simulink model "Laboratorio3CasoA1"  (R2023a)
settings: Solver=VariableStepAuto  StartTime=0.0  StopTime=3/Frecuencia  RelTol=1e-3
undefined symbols (not defined in the file): LCarga, LLinea, RCarga, RLLinea, VSPeak, VSRms
libraries: spsPowerLib x6, spsSeriesRLCBranchLib x4, spsMultimeterLib x2, spsLinearTransformerLib x2, spsACVoltageSourceLib x2, spspowerguiLib x1
settings Model: Creator=mluser  LastModifiedBy=USUARIO
settings OptimizationCC: ReuseModelBlockBuffer=off

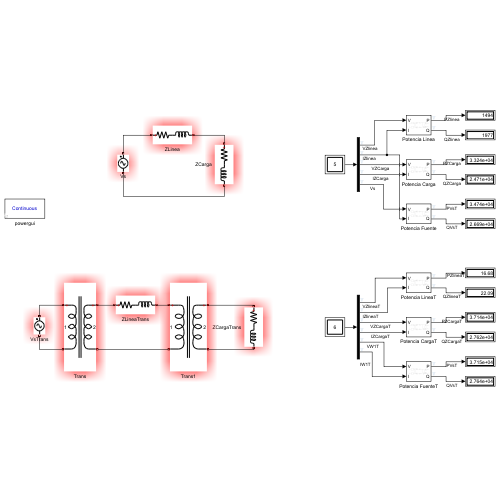
[thumbnail: Simulink's stored preview of the top-level diagram]
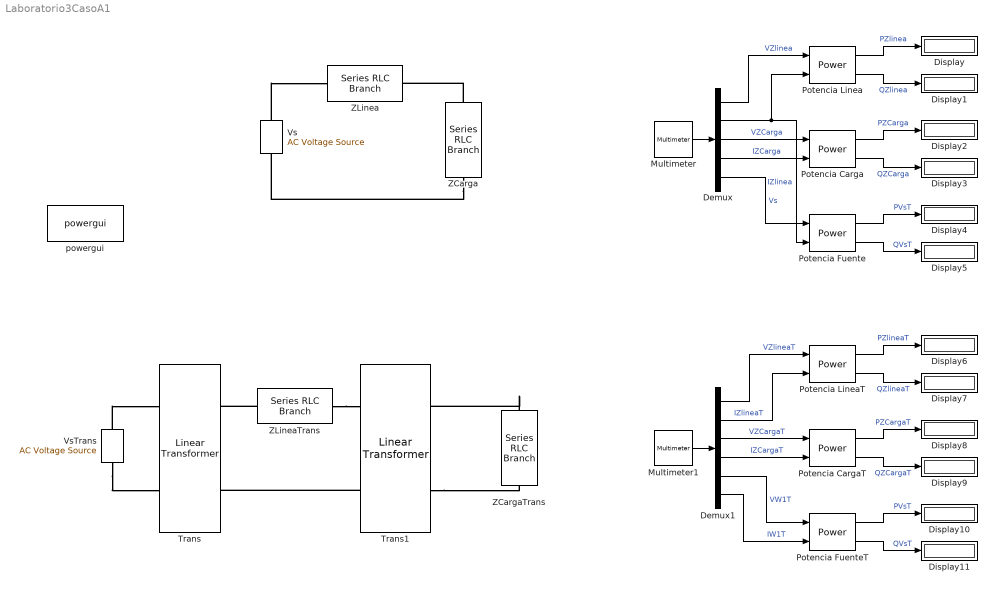
== system Laboratorio3CasoA1 ==
  Demux : Demux  Outputs=5
  Demux1 : Demux  Outputs=6
  Display{,1..11} (12 alike) : Display
  Multimeter : spsMultimeterLib/Multimeter  L=24  sel=[3 13 1 11 9]  yselected={}  Gain=[1 1 1 1 1]  OutputType=Complex  PlotAtSimulationStop=off  PhasorSimulation=off
  Multimeter1 : spsMultimeterLib/Multimeter  L=24  sel=[4 14 2 12 5 15]  yselected={}  Gain=[1 1 1 1 1 1]  OutputType=Complex  PlotAtSimulationStop=off  PhasorSimulation=off
  Potencia Carga : spsPowerLib/Power  Freq=Frecuencia  Vinit=[1, 0]  Iinit=[1, 0]  Ts=0
  Potencia CargaT : spsPowerLib/Power  Freq=Frecuencia  Vinit=[1, 0]  Iinit=[1, 0]  Ts=0
  Potencia Fuente : spsPowerLib/Power  Freq=Frecuencia  Vinit=[1, 0]  Iinit=[1, 0]  Ts=0
  Potencia FuenteT : spsPowerLib/Power  Freq=Frecuencia  Vinit=[1, 0]  Iinit=[1, 0]  Ts=0
  Potencia Linea : spsPowerLib/Power  Freq=Frecuencia  Vinit=[1, 0]  Iinit=[1, 0]  Ts=0
  Potencia LineaT : spsPowerLib/Power  Freq=Frecuencia  Vinit=[1, 0]  Iinit=[1, 0]  Ts=0
  Trans : spsLinearTransformerLib/Linear Transformer  UNITS=SI  NominalPower=[ 250e6 60 ]  winding1=[VSRms 0 0]  winding2=[VSRms*10 0 0]  ThreeWindings=off  winding3=[3.15e+05 0.7938 0.084225]  RmLm=[1.0804e+10 286600]  Measurements=All voltages and currents  DataType=on
  Trans1 : spsLinearTransformerLib/Linear Transformer  UNITS=SI  NominalPower=[ 250e6 60 ]  winding1=[VSRms*10 0 0]  winding2=[VSRms 0 0]  ThreeWindings=off  winding3=[3.15e+05 0.7938 0.084225]  RmLm=[1.0804e+10 286600]  Measurements=All voltages and currents  DataType=on
  Vs : spsACVoltageSourceLib/AC Voltage Source  Amplitude=VSPeak  Phase=0  Frequency=60  SampleTime=0  Measurements=Voltage  BusType=swing  Pref=10e3  Qref=0  Qmin=-inf  Qmax=+inf
  VsTrans : spsACVoltageSourceLib/AC Voltage Source  Amplitude=VSPeak  Phase=0  Frequency=60  SampleTime=0  Measurements=Voltage  BusType=swing  Pref=10e3  Qref=0  Qmin=-inf  Qmax=+inf
  ZCarga : spsSeriesRLCBranchLib/Series RLC Branch  LConnTagsString=__new0  RConnTagsString=__new0  BranchType=RL  Resistance=RCarga  Inductance=LCarga  SetiL0=off  InitialCurrent=0  Capacitance=0  Setx0=off  InitialVoltage=0  Measurements=Branch voltage and current
  ZCargaTrans : spsSeriesRLCBranchLib/Series RLC Branch  LConnTagsString=__new0  RConnTagsString=__new0  BranchType=RL  Resistance=RCarga  Inductance=LCarga  SetiL0=off  InitialCurrent=0  Capacitance=0  Setx0=off  InitialVoltage=0  Measurements=Branch voltage and current
  ZLinea : spsSeriesRLCBranchLib/Series RLC Branch  LConnTagsString=__new0  RConnTagsString=__new0  BranchType=RL  Resistance=RLLinea  Inductance=LLinea  SetiL0=off  InitialCurrent=0  Capacitance=0  Setx0=off  InitialVoltage=0  Measurements=Branch voltage and current
  ZLineaTrans : spsSeriesRLCBranchLib/Series RLC Branch  LConnTagsString=__new0  RConnTagsString=__new0  BranchType=RL  Resistance=RLLinea  Inductance=LLinea  SetiL0=off  InitialCurrent=0  Capacitance=0  Setx0=off  InitialVoltage=0  Measurements=Branch voltage and current
  powergui : spspowerguiLib/powergui  Priority=1  SimulationMode=Continuous  SampleTime=50e-6  frequency=60  Iterations=50  frequencyindice=60  Pbase=100e6  ErrMax=1e-4  UnitsV=kV  UnitsW=MW  buscounter=0  FunctionMessages=off  echomessages=off  EnableUseOfTLC=off  CurrentSourceSwitches=off  DisableSnubberDevices=off  DisableRonSwitches=off  DisableVfSwitches=off  DisplayEquations=off  AutomaticDiscreteSolvers=off  SolverType=Tustin/Backward Euler (TBE)  Interpol=off  ExternalGateDelay=off  methode=off  Ts=100  x0status=blocks  SPID=on  SwTol=0  HookPort=off  NonlinearTolerance=1e-4  nMaxIteration=100  ContinueOnMaxIteration=off  RestoreLinks=warning  ResistiveCurrentMeasurement=off  Frange=[0:2:500]  Ylog=off  Xlog=on  ShowGrid=off  save=off  variable=ZData  structure=0  ZoomFFT=off  StartTime=0.0  cycles=1  DisplayStyle=1  fundamental=60  FreqAxis=off  MaxFrequency=1000  frequencyindicesteady=1  RmsSteady=1  display=off
  wires:
  Multimeter/1 -> Demux/1
  Demux/3 -> Potencia Carga/1  "VZCarga"
  Demux/4 -> Potencia Carga/2  "IZCarga"
  Demux/2 -> Potencia Fuente/2, Potencia Linea/2  "IZlinea"
  Demux/1 -> Potencia Linea/1  "VZlinea"
  Potencia Linea/1 -> Display/1  "PZlinea"
  Potencia Linea/2 -> Display1/1  "QZlinea"
  Potencia Carga/1 -> Display2/1  "PZCarga"
  Potencia Carga/2 -> Display3/1  "QZCarga"
  Demux/5 -> Potencia Fuente/1  "Vs"
  Potencia Fuente/1 -> Display4/1  "PVsT"
  Potencia Fuente/2 -> Display5/1  "QVsT"
  Potencia CargaT/1 -> Display8/1  "PZCargaT"
  Demux1/5 -> Potencia FuenteT/1  "VW1T"
  Potencia CargaT/2 -> Display9/1  "QZCargaT"
  Potencia FuenteT/2 -> Display11/1  "QVsT"
  Potencia LineaT/1 -> Display6/1  "PZlineaT"
  Demux1/3 -> Potencia CargaT/1  "VZCargaT"
  Demux1/2 -> Potencia LineaT/2  "IZlineaT"
  Demux1/4 -> Potencia CargaT/2  "IZCargaT"
  Multimeter1/1 -> Demux1/1
  Potencia LineaT/2 -> Display7/1  "QZlineaT"
  Potencia FuenteT/1 -> Display10/1  "PVsT"
  Demux1/1 -> Potencia LineaT/1  "VZlineaT"
  Demux1/6 -> Potencia FuenteT/2  "IW1T"
  connections:
  ZCarga/LConn1 -- ZLinea/RConn1
  ZCarga/RConn1 -- Vs/LConn1
  Vs/RConn1 -- ZLinea/LConn1
  VsTrans/RConn1 -- Trans/LConn1
  VsTrans/LConn1 -- Trans/LConn2
  ZLineaTrans/LConn1 -- Trans/RConn1
  ZLineaTrans/RConn1 -- Trans1/LConn1
  ZCargaTrans/LConn1 -- Trans1/RConn1
  Trans1/RConn2 -- ZCargaTrans/RConn1
  Trans1/LConn2 -- Trans/RConn2
